simulink model "TST_AdvancedStateflowLoops"  (Simulink 7.4)
settings: Solver=FixedStepDiscrete  StartTime=0.0  StopTime=10.0  FixedStep=0.02  RelTol=1e-3
settings Model: Creator=kharthforeign  LastModifiedBy=kharthforeign  BufferReuse=off
settings DataIOCC: SaveOutput=off  SignalLogging=off  SaveTime=off
settings OptimizationCC: BlockReduction=off  ConditionallyExecuteInputs=off  OptimizeBlockIOStorage=off  BufferReuse=off  ExpressionFolding=off  LocalBlockOutputs=off  InitFltsAndDblsToZero=on

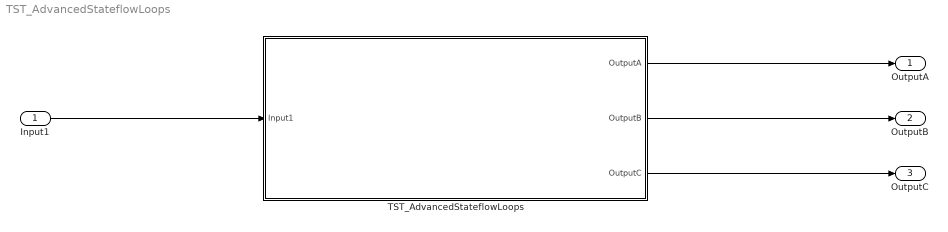
== system TST_AdvancedStateflowLoops ==
  Input1 : Inport  DataType=uint32  OutDataType=fixdt(1, 16)  OutScaling=2^0  OutDataTypeStr=uint32  BusOutputAsStruct=on
  TST_AdvancedStateflowLoops : Subsystem  TreatAsAtomicUnit=on
  OutputA : Outport  PortDimensions=1  DataType=double  OutDataType=fixdt(1, 16)  OutScaling=2^0  OutDataTypeStr=double
  OutputB : Outport  Port=2  PortDimensions=1  DataType=double  OutDataType=Enum: DIL_VmmGsFcsCommandsMessage_LatApModeCmd  OutDataTypeStr=double
  OutputC : Outport  Port=3  PortDimensions=1  DataType=double  OutDataType=fixdt(1, 16)  OutScaling=2^0  OutDataTypeStr=double
  wires:
  Input1/1 -> TST_AdvancedStateflowLoops/1(Input1)
  TST_AdvancedStateflowLoops/1(OutputA) -> OutputA/1
  TST_AdvancedStateflowLoops/2(OutputB) -> OutputB/1
  TST_AdvancedStateflowLoops/3(OutputC) -> OutputC/1

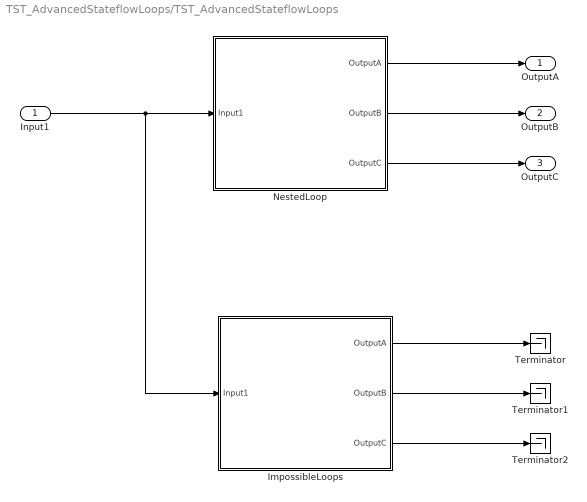
== system TST_AdvancedStateflowLoops/TST_AdvancedStateflowLoops ==
  Input1 : Inport  DataType=uint32  OutDataType=fixdt(1, 16)  OutScaling=2^0  OutDataTypeStr=uint32  BusOutputAsStruct=on
  ImpossibleLoops : Stateflow chart
  NestedLoop : Stateflow chart
  Terminator : Terminator
  Terminator1 : Terminator
  Terminator2 : Terminator
  OutputA : Outport  PortDimensions=1  DataType=double  OutDataType=fixdt(1, 16)  OutScaling=2^0  OutDataTypeStr=double
  OutputB : Outport  Port=2  PortDimensions=1  DataType=double  OutDataType=Enum: DIL_VmmGsFcsCommandsMessage_LatApModeCmd  OutDataTypeStr=double
  OutputC : Outport  Port=3  PortDimensions=1  DataType=double  OutDataType=fixdt(1, 16)  OutScaling=2^0  OutDataTypeStr=double
  wires:
  NestedLoop/1(OutputA) -> OutputA/1
  NestedLoop/2(OutputB) -> OutputB/1
  NestedLoop/3(OutputC) -> OutputC/1
  Input1/1 -> NestedLoop/1(Input1), ImpossibleLoops/1(Input1)
  ImpossibleLoops/1(OutputA) -> Terminator/1
  ImpossibleLoops/2(OutputB) -> Terminator1/1
  ImpossibleLoops/3(OutputC) -> Terminator2/1

== stateflow chart TST_AdvancedStateflowLoops/NestedLoop ==
  note: demonstrate loop nested inside another loop
  (junction 5) -> (junction 6) [order 1] : [A]{OutputA = 1;}%loop1.1
  (junction 5) -> (junction 4) [order 2] : %else to A
  (default) -> (junction 5) : %default
  (junction 6) -> (junction 7) : %loop1.2
  (junction 7) -> (junction 8) [order 2] : %else to B, loop1.3
  (junction 8) -> (junction 5) : %loop1.4
  (junction 7) -> (junction 7) [order 1] : [B]{OutputB = 1;} %loop 2.1
  data: Input1 input uint32; OutputA output double =1; OutputB output double =2; OutputC output double =3; Local local uint32 =0; A local boolean; B local boolean; C local boolean

== stateflow chart TST_AdvancedStateflowLoops/ImpossibleLoops ==
  note: Designing something like this is probably
      | not a good idea!
  note: Even though the graphical presentation doesn not show this
      | well: The second loop (starting with [D] is simply nested
      | inside the first loop (starting at [A]...). Both loops share the [D] transition.
  (junction 29) -> (junction 30) [order 1] : [A]{OutputA = 1;}%loop1.1
  (junction 29) -> (junction 28) [order 2] : %else to A
  (default) -> (junction 29) : %default
  (junction 31) -> (junction 29) [order 1] : [B]{OutputB = 1;}%loop1.3
  (junction 30) -> (junction 31) [order 1] : [D]%loop1.2/2.1
  (junction 31) -> (junction 32) [order 2] : %else to B/loop2.2
  (junction 32) -> (junction 30) [order 1] : [C]{OutputC = 1;}%loop2.3
  (junction 32) -> (junction 33) [order 2] : %else to C
  (junction 30) -> (junction 34) [order 2] : %else to D
  data: Input1 input uint32; OutputA output double =1; OutputB output double =2; OutputC output double =3; Local local uint32 =0; A local boolean; B local boolean; C local boolean; D local boolean
